simulink model "project2"  (R2013a)
settings: Solver=ode45  SolverMode=SingleTasking  StartTime=0.0  StopTime=0.1  RelTol=1e-3
libraries: fl_lib x6, nesl_utility x5, simulink x3
settings Model: Creator=SAEED  LastModifiedBy=KAZEM
settings DataIOCC: SignalLoggingSaveFormat=ModelDataLogs
settings OptimizationCC: BlockReduction=off  BooleanDataType=off
settings DebuggingCC: SaveWithParameterizedLinksMsg=none  SignalResolutionControl=TryResolveAllWithWarning  SolverPrmCheckMsg=none  MultiTaskDSMMsg=warning  MultiTaskCondExecSysMsg=none  StrictBusMsg=None
settings HardwareCC: TargetUnknown=on
settings RTWCC: IncludeERTFirstTime=on

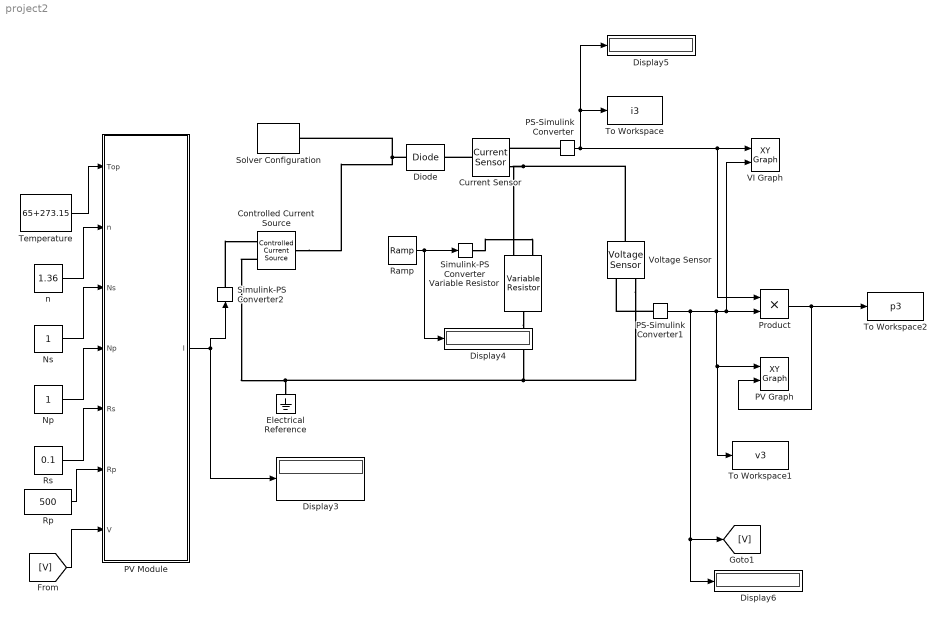
== system project2 ==
  Controlled Current Source : fl_lib/Electrical/Electrical Sources/Controlled Current Source  i_Log=off  v_Log=off  LocalVarNames=|i|v  LocalVarDescs=|i|v  LocalVarLogging=[0 0]
  Current Sensor : fl_lib/Electrical/Electrical Sensors/Current Sensor  i1_Log=off  v1_Log=off  LocalVarNames=|i1|v1  LocalVarDescs=|i1|v1  LocalVarLogging=[0 0]
  Diode : fl_lib/Electrical/Electrical Elements/Diode  Vf=0.6 V  Ron=0.3 Ohm  Goff=1e-8 1/Ohm  i_Log=off  v_Log=off  LocalVarNames=|i|v  LocalVarDescs=|i|v  LocalVarLogging=[0 0]
  Display{3..6} (4 alike) : Display
  Electrical Reference : fl_lib/Electrical/Electrical Elements/Electrical Reference  i_Log=off  LocalVarNames=|i  LocalVarDescs=|i  LocalVarLogging=0
  Np : Constant
  Ns : Constant
  PS-Simulink Converter : nesl_utility/PS-Simulink Converter  PhysicalDomain=network_engine_domain  SubClassName=ps_output  LeftPortType=input  RightPortType=output  PseudoPeriodic=off  Frequencies=[]  Unit=1  AffineConversion=off
  PS-Simulink Converter1 : nesl_utility/PS-Simulink Converter  PhysicalDomain=network_engine_domain  SubClassName=ps_output  LeftPortType=input  RightPortType=output  PseudoPeriodic=off  Frequencies=[]  Unit=1  AffineConversion=off
  PV Graph : simulink/Sinks/XY Graph  xmin=0  xmax=25  ymin=0  ymax=40  st=-1
  PV Module : Subsystem
  Product : Product
  Ramp : simulink/Sources/Ramp  slope=7000  start=0  X0=0
  Rp : Constant  Value=500
  Rs : Constant  Value=0.1
  Simulink-PS Converter : nesl_utility/Simulink-PS Converter  PhysicalDomain=network_engine_domain  SubClassName=ps_input  LeftPortType=input  RightPortType=output  PseudoPeriodic=off  Frequencies=[]  NoiseDistribution=none  NoiseParameters=[]  Unit=1  AffineConversion=off  InputFiltering=off  SimscapeFilterOrder=1  InputFilterTimeConstant=0.001  UdotUserProvided=1
  Simulink-PS Converter2 : nesl_utility/Simulink-PS Converter  PhysicalDomain=network_engine_domain  SubClassName=ps_input  LeftPortType=input  RightPortType=output  PseudoPeriodic=off  Frequencies=[]  NoiseDistribution=none  NoiseParameters=[]  Unit=1  AffineConversion=off  InputFiltering=off  SimscapeFilterOrder=1  InputFilterTimeConstant=0.001  UdotUserProvided=1
  Solver Configuration : nesl_utility/Solver Configuration  PhysicalDomain=network_engine_domain  SubClassName=solver  LeftPortType=input  RightPortType=generic  Accelerate=off  Tones=[]  Harmonics=[]  SimulateNoise=off  Profile=off  UseLocalSampling=off  EnableSwitchedLinearOptims=on  FrequencyDomain=off  UseCCode=off  UseNewInitialization=off  DoDC=off  ResidualTolerance=1e-8  UseLocalSolver=on  LocalSolverChoice=NE_BACKWARD_EULER_ADVANCER  LocalSolverSampleTime=0.0001  DoFixedCost=on  MaxNonlinIter=3  MaxModeIter=2  LinearAlgebra=Sparse  DelaysMemoryBudget=1024
  Temperature : Constant  Value=65+273.15
  To Workspace : ToWorkspace  VariableName=i3  SampleTime=0.00001
      settings: Decimation=2
  To Workspace1 : ToWorkspace  VariableName=v3  SampleTime=0.00001
      settings: Decimation=2
  To Workspace2 : ToWorkspace  VariableName=p3  SampleTime=0.00001
      settings: Decimation=2
  VI Graph : simulink/Sinks/XY Graph  xmin=0  xmax=10  ymin=0  ymax=30  st=-1
  Variable Resistor : fl_lib/Electrical/Electrical Elements/Variable Resistor  Rmin=0 Ohm  i_Log=off  v_Log=off  LocalVarNames=|i|v  LocalVarDescs=|i|v  LocalVarLogging=[0 0]
  Voltage Sensor : fl_lib/Electrical/Electrical Sensors/Voltage Sensor  i1_Log=off  v1_Log=off  LocalVarNames=|i1|v1  LocalVarDescs=|i1|v1  LocalVarLogging=[0 0]
  n : Constant  Value=1.36
  wires:
  PV Module/1(I) -> Simulink-PS Converter2/1, Display3/1
  n/1 -> PV Module/2(n)
  Ns/1 -> PV Module/3(Ns)
  Np/1 -> PV Module/4(Np)
  Rp/1 -> PV Module/6(Rp)
  Temperature/1 -> PV Module/1(Top)
  Rs/1 -> PV Module/5(Rs)
  Ramp/1 -> Simulink-PS Converter/1, Display4/1
  [V] -> PV Module/7(V)
  PS-Simulink Converter/1 -> To Workspace/1, Display5/1, Product/1, VI Graph/1
  Product/1 -> To Workspace2/1, PV Graph/2
  PS-Simulink Converter1/1 -> Display6/1, [V], Product/2, VI Graph/2, To Workspace1/1, PV Graph/1
  connections:
  Diode/LConn1 -- Controlled Current Source/LConn1 -- Solver Configuration/RConn1
  Current Sensor/LConn1 -- Diode/RConn1
  PS-Simulink Converter/LConn1 -- Current Sensor/RConn1
  Voltage Sensor/RConn2 -- Variable Resistor/RConn1 -- Controlled Current Source/RConn2 -- Electrical Reference/LConn1
  Current Sensor/RConn2 -- Voltage Sensor/LConn1 -- Variable Resistor/LConn2
  Simulink-PS Converter/RConn1 -- Variable Resistor/LConn1
  PS-Simulink Converter1/LConn1 -- Voltage Sensor/RConn1
  Simulink-PS Converter2/RConn1 -- Controlled Current Source/RConn1

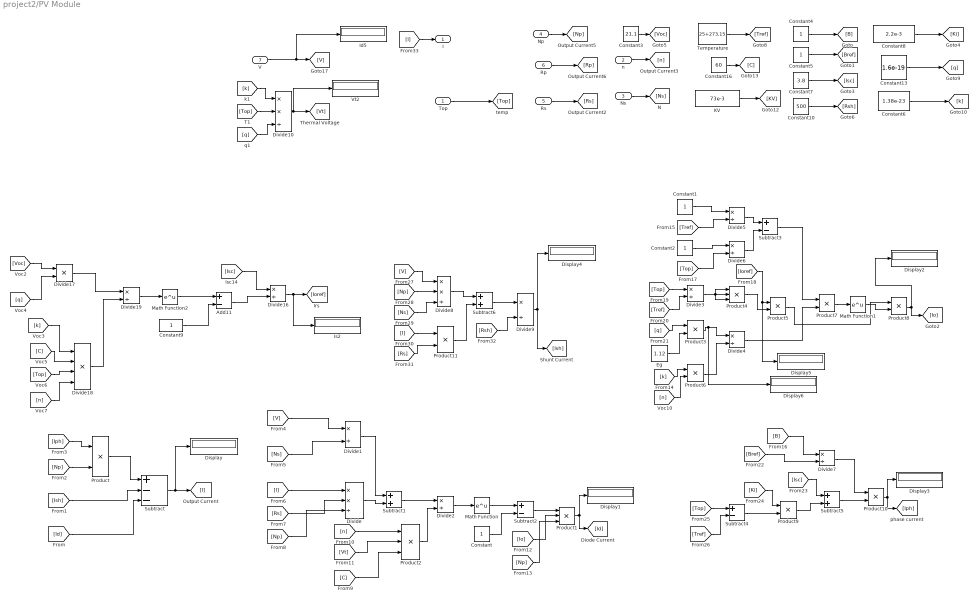
== system project2/PV Module ==
  Top : Inport
  n : Inport  Port=2
  Ns : Inport  Port=3
  Np : Inport  Port=4
  Rs : Inport  Port=5
  Rp : Inport  Port=6
  V : Inport  Port=7
  Add11 : Sum  Inputs=+-
  Constant{,1..2,4..5,9} (6 alike) : Constant
  Constant10 : Constant  Value=500
  Constant13 : Constant  Value=1.6e-19
  Constant16 : Constant  Value=60
  Constant3 : Constant  Value=21.1
  Constant6 : Constant  Value=1.38e-23
  Constant7 : Constant  Value=3.8
  Constant8 : Constant  Value=2.2e-3
  Display{,1..6} (7 alike) : Display
  Divide : Product  Inputs=**/
  Divide{1..7,9,16,19} (10 alike) : Product  Inputs=*/
  Divide10 : Product  Inputs=**/
  Divide17 : Product  Inputs=**
  Divide18 : Product  Inputs=****
  Divide8 : Product  Inputs=**/
  Eg : Constant  Value=1.12
  Id5 : Display
  Is2 : Display
  KV : Constant  Value=73e-3
  Math Function : Math  SaturateOnIntegerOverflow=on
  Math Function1 : Math  SaturateOnIntegerOverflow=on
  Math Function2 : Math  SaturateOnIntegerOverflow=on
  Product{,3,5..11} (9 alike) : Product
  Product1 : Product  Inputs=3
  Product2 : Product  Inputs=3
  Product4 : Product  Inputs=3
  Subtract : Sum  Inputs=+--
  Subtract1 : Sum
  Subtract2 : Sum  Inputs=+-
  Subtract3 : Sum  Inputs=+-
  Subtract4 : Sum  Inputs=+-
  Subtract5 : Sum
  Subtract6 : Sum
  Temperature : Constant  Value=25+273.15
  Vt2 : Display
      settings: Format=long_e
  I : Outport
  wires:
  [Id] -> Subtract/3
  [Ish] -> Subtract/2
  Product/1 -> Subtract/1
  Divide1/1 -> Subtract1/1
  Divide/1 -> Subtract1/2
  Subtract1/1 -> Divide2/1
  Product2/1 -> Divide2/2
  Divide2/1 -> Math Function/1
  Math Function/1 -> Subtract2/1
  Constant/1 -> Subtract2/2
  Subtract2/1 -> Product1/1
  Product1/1 -> [Id], Display1/1
  [Ns] -> Divide1/2
  [I] -> Divide/1
  [Rs] -> Divide/2
  [n] -> Product2/1
  [C] -> Product2/3
  [Vt] -> Product2/2
  [Io] -> Product1/2
  [Np] -> Product1/3
  Divide3/1 -> Product4/3, Product4/1, Product4/2
  Product4/1 -> Product5/2
  Product3/1 -> Display6/1, Divide4/1
  Product6/1 -> Divide4/2
  Divide6/1 -> Subtract3/2
  Subtract3/1 -> Product7/1
  Divide4/1 -> Product7/2
  Product7/1 -> Math Function1/1
  Math Function1/1 -> Product8/2
  Product5/1 -> Product8/1
  Product8/1 -> [Io], Display2/1
  Constant1/1 -> Divide5/1
  [Tref] -> Divide5/2
  [Top] -> Divide6/2
  Constant2/1 -> Divide6/1
  [Ioref] -> Display5/1, Product5/1
  [Top] -> Divide3/1
  [Tref] -> Divide3/2
  [q] -> Product3/1
  Eg/1 -> Product3/2
  [k] -> Product6/1
  [n] -> Product6/2
  Product10/1 -> Display3/1, [Iph]
  Subtract4/1 -> Product9/2
  Product9/1 -> Subtract5/2
  Subtract5/1 -> Product10/2
  Divide7/1 -> Product10/1
  [B] -> Divide7/1
  [Top] -> Subtract4/1
  [Tref] -> Subtract4/2
  [Bref] -> Divide7/2
  [Isc] -> Subtract5/1
  [Ki] -> Product9/1
  Divide8/1 -> Subtract6/1
  Product11/1 -> Subtract6/2
  Subtract6/1 -> Divide9/1
  Divide9/1 -> Display4/1, [Ish]
  [V] -> Divide8/1
  [Np] -> Divide8/2
  [Ns] -> Divide8/3
  [I] -> Product11/1
  [Rs] -> Product11/2
  n/1 -> [n]
  Ns/1 -> [Ns]
  Np/1 -> [Np]
  Constant7/1 -> [Isc]
  Constant10/1 -> [Rsh]
  Temperature/1 -> [Tref]
  Constant13/1 -> [q]
  Constant6/1 -> [k]
  Constant8/1 -> [Ki]
  Constant16/1 -> [C]
  [V] -> Divide1/1
  Top/1 -> [Top]
  Rs/1 -> [Rs]
  [I] -> I/1
  Divide5/1 -> Subtract3/1
  [Iph] -> Product/1
  [Np] -> Product/2
  Constant5/1 -> [Bref]
  Constant3/1 -> [Voc]
  Constant4/1 -> [B]
  [k] -> Divide10/1
  Divide10/1 -> [Vt], Vt2/1
  [Top] -> Divide10/2
  [q] -> Divide10/3
  Constant9/1 -> Add11/2
  [q] -> Divide17/2
  Divide16/1 -> [Ioref], Is2/1
  Math Function2/1 -> Add11/1
  Add11/1 -> Divide16/2
  [k] -> Divide18/1
  [n] -> Divide18/4
  Divide17/1 -> Divide19/1
  Divide18/1 -> Divide19/2
  [Voc] -> Divide17/1
  [Top] -> Divide18/3
  [C] -> Divide18/2
  Divide19/1 -> Math Function2/1
  [Isc] -> Divide16/1
  [Np] -> Divide/3
  Rp/1 -> [Rp]
  KV/1 -> [KV]
  V/1 -> [V], Id5/1
  [Rsh] -> Divide9/2
  Subtract/1 -> Display/1, [I]
